simulink model "DC_Motor_Position_Control"  (Simulink 8.9)
settings: Solver=ode45  StartTime=0.0  StopTime=5.0  RelTol=1e-3  EnableMultiTasking=on
libraries: simulink x1
settings Model: Creator=a.tahir.uetlhr  LastModifiedBy=abxis
settings OptimizationCC: InitFltsAndDblsToZero=on
settings DebuggingCC: SaveWithParameterizedLinksMsg=none  SignalResolutionControl=TryResolveAllWithWarning  SolverPrmCheckMsg=warning  MultiTaskDSMMsg=warning  MultiTaskCondExecSysMsg=none  FcnCallInpInsideContextMsg=error  StateNameClashWarn=none
settings GRTTargetCC: TargetFcnLib=ansi_tfl_tmw.mat  GeneratePreprocessorConditionals=Use local settings

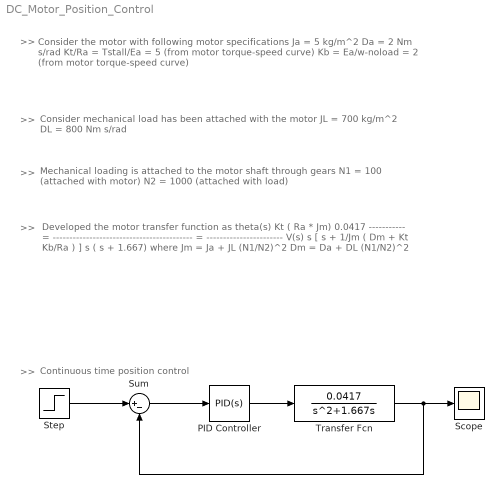
== system DC_Motor_Position_Control ==
  note: >>
  note: Continuous time position control
  note: >>
  note: >>
  note: >>
  note: >>
  note: Developed the motor transfer function as
      |
      | theta(s) Kt ( Ra * Jm) 0.0417
      | ----------- = ------------------------------------------ = -----------------------
      | V(s) s [ s + 1/Jm ( Dm + Kt Kb/Ra ) ] s ( s + 1.667)
      |
      | where
      | Jm = Ja + JL (N1/N2)^2
      | Dm = Da + DL (N1/N2)^2
  note: Mechanical loading is attached to the motor shaft through gears
      | N1 = 100 (attached with motor)
      | N2 = 1000 (attached with load)
  note: Consider mechanical load has been attached with the motor
      | JL = 700 kg/m^2
      | DL = 800 Nm s/rad
  note: Consider the motor with following motor specifications
      | Ja = 5 kg/m^2
      | Da = 2 Nm s/rad
      | Kt/Ra = Tstall/Ea = 5 (from motor torque-speed curve)
      | Kb = Ea/w-noload = 2 (from motor torque-speed curve)
  PID Controller : simulink/Continuous/PID Controller  Controller=PID  TimeDomain=Continuous-time  SampleTime=-1  IntegratorMethod=Forward Euler  FilterMethod=Forward Euler  Form=Parallel  UseFilter=on  ControllerParametersSource=internal  P=600  I=10  D=400  N=102.168277238528  InitialConditionSource=internal  InitialConditionForIntegrator=0  InitialConditionForFilter=0  ExternalReset=none  LimitOutput=off  UpperSaturationLimit=inf  LowerSaturationLimit=-inf  LinearizeAsGain=on  AntiWindupMode=none  Kb=1  TrackingMode=off  Kt=1  PParamMin=[]  PParamMax=[]  IParamMin=[]  IParamMax=[]  DParamMin=[]  DParamMax=[]  NParamMin=[]  NParamMax=[]  KbParamMin=[]  KbParamMax=[]  KtParamMin=[]  KtParamMax=[]  POutMin=[]  POutMax=[]  IOutMin=[]  IOutMax=[]  DOutMin=[]  DOutMax=[]  NOutMin=[]  NOutMax=[]  KbOutMin=[]  KbOutMax=[]  KtOutMin=[]  KtOutMax=[]  IntegratorOutMin=[]  IntegratorOutMax=[]  FilterOutMin=[]  FilterOutMax=[]  SumOutMin=[]  SumOutMax=[]  SumI1OutMin=[]  SumI1OutMax=[]  SumI2OutMin=[]  SumI2OutMax=[]  SumI3OutMin=[]  SumI3OutMax=[]  SumDOutMin=[]  SumDOutMax=[]  SaturationOutMin=[]  SaturationOutMax=[]  IntegratorContinuousStateAttributes=''  IntegratorStateMustResolveToSignalObject=off  IntegratorRTWStateStorageClass=Auto  FilterContinuousStateAttributes=''  FilterStateMustResolveToSignalObject=off  FilterRTWStateStorageClass=Auto  DifferentiatorICPrevScaledInput=0  DifferentiatorOutMin=[]  DifferentiatorOutMax=[]  InitialConditionSetting=State (most efficient)
  Scope : Scope
  Step : Step  Time=0  SampleTime=0
  Sum : Sum  Inputs=|+-
  Transfer Fcn : TransferFcn  Numerator=[0.0417]  Denominator=[1 1.667 0]
  wires:
  Step/1 -> Sum/1
  Transfer Fcn/1 -> Scope/1, Sum/2
  Sum/1 -> PID Controller/1
  PID Controller/1 -> Transfer Fcn/1
